simulink model "Fig418"  (R2014b)
settings: Solver=FixedStepDiscrete  StartTime=0.0  StopTime=.02  RelTol=1e-3
libraries: commrandsrc2 x1
settings Model: Creator=Silage  LastModifiedBy=Silage
settings DataIOCC: SignalLoggingSaveFormat=ModelDataLogs
settings OptimizationCC: ExpressionDepthLimit=2147483647
settings DebuggingCC: UnderspecifiedInitializationDetection=Classic  MergeDetectMultiDrivingBlocksExec=none  FcnCallInpInsideContextMsg=EnableAllAsWarning  StateNameClashWarn=warning
settings GRTTargetCC: CombineOutputUpdateFcns=off  GRTInterface=on

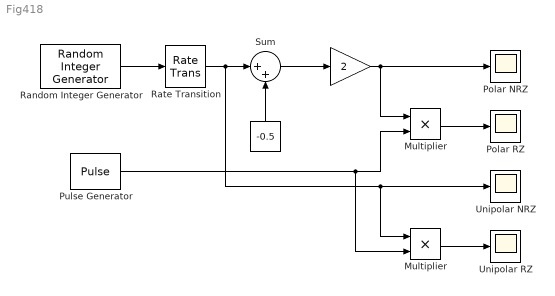
== system Fig418 ==
  " " : Constant  Value=-0.5
  "   " : Gain  Gain=2
  Multiplier : Product  RndMeth=Zero
  "Multiplier " : Product  RndMeth=Zero
  Polar NRZ : Scope
      settings: YMin=-1.5  YMax=1.5
  Polar RZ : Scope
      settings: YMin=-1.5  YMax=1.5
  Pulse Generator : DiscretePulseGenerator  Period=50  PulseWidth=25  SampleTime=2e-5
  Random Integer Generator : commrandsrc2/Random Integer Generator  mul=2  seed=randseed  Ts=1e-3  frameBased=off  sampPerFrame=1  orient=on  outDataType=double
  Rate Transition : RateTransition  OutPortSampleTime=2e-5
  Sum : Sum  Inputs=|++
  Unipolar NRZ : Scope
      settings: YMin=-1.5  YMax=1.5  SaveName=ScopeData2
  Unipolar RZ : Scope
      settings: YMin=-1.5  YMax=1.5  SaveName=ScopeData3
  wires:
  Random Integer Generator/1 -> Rate Transition/1
  Rate Transition/1 -> Sum/1, "Multiplier "/1, Unipolar NRZ/1
  " "/1 -> Sum/2
  Sum/1 -> "   "/1
  "   "/1 -> Polar NRZ/1, Multiplier/1
  Multiplier/1 -> Polar RZ/1
  Pulse Generator/1 -> Multiplier/2, "Multiplier "/2
  "Multiplier "/1 -> Unipolar RZ/1
